simulink model "Half_Car_Model"  (R2024b)
settings: Solver=VariableStepAuto  StartTime=0.0  StopTime=4.5  RelTol=1e-3
model workspace (MAT data in the model file):
  I_yy = Simulink.Parameter
  I_yy.Value = 76.97
  I_yy.Complexity = 'real'
  I_yy.Dimensions = [1 1]
  I_yy.Description = 'Pitch moment of inertia (from solidworks TG19)'
  I_yy.DataType = 'auto'
  I_yy.DocUnits = 'kg/m/m'
  L = Simulink.Parameter
  L.Value = 1.49
  L.Complexity = 'real'
  L.Dimensions = [1 1]
  L.Description = 'wheelbase TG19 solidworks'
  L.DataType = 'auto'
  L.DocUnits = 'm'
  L_F = Simulink.Parameter
  L_F.Value = 0.91
  L_F.Complexity = 'real'
  L_F.Dimensions = [1 1]
  L_F.Description = 'distance from COM to front axle'
  L_F.DataType = 'auto'
  L_F.DocUnits = 'm'
  L_R = Simulink.Parameter
  L_R.Value = 0.58
  L_R.Complexity = 'real'
  L_R.Dimensions = [1 1]
  L_R.Description = 'distance from COM to rear axle'
  L_R.DataType = 'auto'
  L_R.DocUnits = 'm'
  c_Fs = Simulink.Parameter
  c_Fs.Value = 237.5
  c_Fs.Complexity = 'real'
  c_Fs.Dimensions = [1 1]
  c_Fs.Description = 'Shock damping from TG19 Spring Sheet'
  c_Fs.DataType = 'auto'
  c_Fs.DocUnits = 'kg/s'
  c_Fw = Simulink.Parameter
  c_Fw.Value = 1500
  c_Fw.Complexity = 'real'
  c_Fw.Dimensions = [1 1]
  c_Fw.Description = 'Tyre damping from Internet Value'
  c_Fw.DataType = 'auto'
  c_Fw.DocUnits = 'kg/s'
  c_Rs = Simulink.Parameter
  c_Rs.Value = 237.5
  c_Rs.Complexity = 'real'
  c_Rs.Dimensions = [1 1]
  c_Rs.Description = 'Shock damping from TG19 Spring Sheet'
  c_Rs.DataType = 'auto'
  c_Rs.DocUnits = 'kg/s'
  c_Rw = Simulink.Parameter
  c_Rw.Value = 1500
  c_Rw.Complexity = 'real'
  c_Rw.Dimensions = [1 1]
  c_Rw.Description = 'Tyre damping from Internet Value'
  c_Rw.DataType = 'auto'
  c_Rw.DocUnits = 'kg/s'
  gLong = Simulink.Parameter
  gLong.Value = 0
  gLong.Complexity = 'real'
  gLong.Dimensions = [1 1]
  gLong.Description = 'Longitudinal acceleration of car'
  gLong.DataType = 'auto'
  gLong.DocUnits = 'm/s/s'
  h = Simulink.Parameter
  h.Value = 0.51
  h.Complexity = 'real'
  h.Dimensions = [1 1]
  h.Description = 'height of com above ground at ride height (guessed)'
  h.DataType = 'auto'
  h.DocUnits = 'm'
  k_Fs = Simulink.Parameter
  k_Fs.Value = 3159.177
  k_Fs.Complexity = 'real'
  k_Fs.Dimensions = [1 1]
  k_Fs.Description = 'Shock Spring Rate from TG19 Shocks sheet (wheel rate value)'
  k_Fs.DataType = 'double'
  k_Fs.DocUnits = 'N/m'
  k_Fw = Simulink.Parameter
  k_Fw.Value = 30992
  k_Fw.Complexity = 'real'
  k_Fw.Dimensions = [1 1]
  k_Fw.Description = 'Tire Spring Stiffness (from internet value)'
  k_Fw.DataType = 'auto'
  k_Fw.DocUnits = 'N/m'
  k_Rs = Simulink.Parameter
  k_Rs.Value = 3159.177
  k_Rs.Complexity = 'real'
  k_Rs.Dimensions = [1 1]
  k_Rs.Description = 'Shock Spring Rate from TG19 Shocks sheet (wheel rate value)'
  k_Rs.DataType = 'double'
  k_Rs.DocUnits = 'N/m'
  k_Rw = Simulink.Parameter
  k_Rw.Value = 30992
  k_Rw.Complexity = 'real'
  k_Rw.Dimensions = [1 1]
  k_Rw.Description = 'Tire Spring Stiffness (from internet value)'
  k_Rw.DataType = 'auto'
  k_Rw.DocUnits = 'N/m'
  m_F = Simulink.Parameter
  m_F.Value = 27.27
  m_F.Complexity = 'real'
  m_F.Dimensions = [1 1]
  m_F.Description = 'Unsprung front axle mass'
  m_F.DataType = 'auto'
  m_F.DocUnits = 'kg'
  m_R = Simulink.Parameter
  m_R.Value = 27.7
  m_R.Complexity = 'real'
  m_R.Dimensions = [1 1]
  m_R.Description = 'unsprung rear axle mass from TG19 Shock sheet
    | = 30*2'
  m_R.DataType = 'auto'
  m_R.DocUnits = 'kg'
  m_s = Simulink.Parameter
  m_s.Value = 129
  m_s.Complexity = 'real'
  m_s.Dimensions = [1 1]
  m_s.Description = 'sprung mass from TG19 Shock sheet without 60kg driver'
  m_s.DataType = 'auto'
  m_s.DocUnits = 'kg'
  v = Simulink.Parameter
  v.Value = 11
  v.Complexity = 'real'
  v.Dimensions = [1 1]
  v.Description = 'initial velocity of car (40kph)'
  v.DataType = 'auto'
  v.DocUnits = 'm/s'
values from neighbouring files (symbols this model uses):
  L_F = mdlWks.getVariable('L_F').Value    [HCM_Animation.m]
  L_R = mdlWks.getVariable('L_R').Value    [HCM_Animation.m]
  v = -(amp/2)*freq*cos(freq*t)*.0254    [BumpBump.m]
libraries: simulink x1
settings Model: Creator=arnav  LastModifiedBy=arnav
settings RTWCC: GPUComputeCapability=3.5

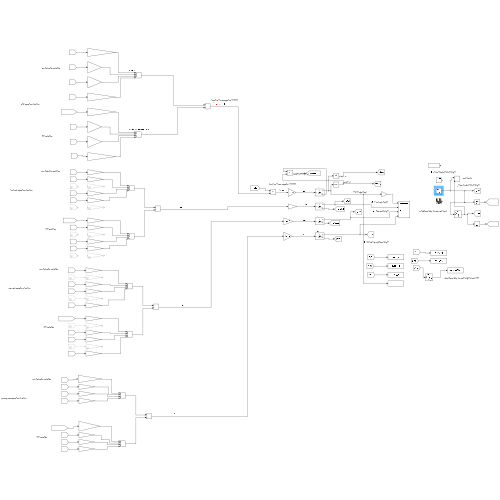
[thumbnail: Simulink's stored preview of the top-level diagram]
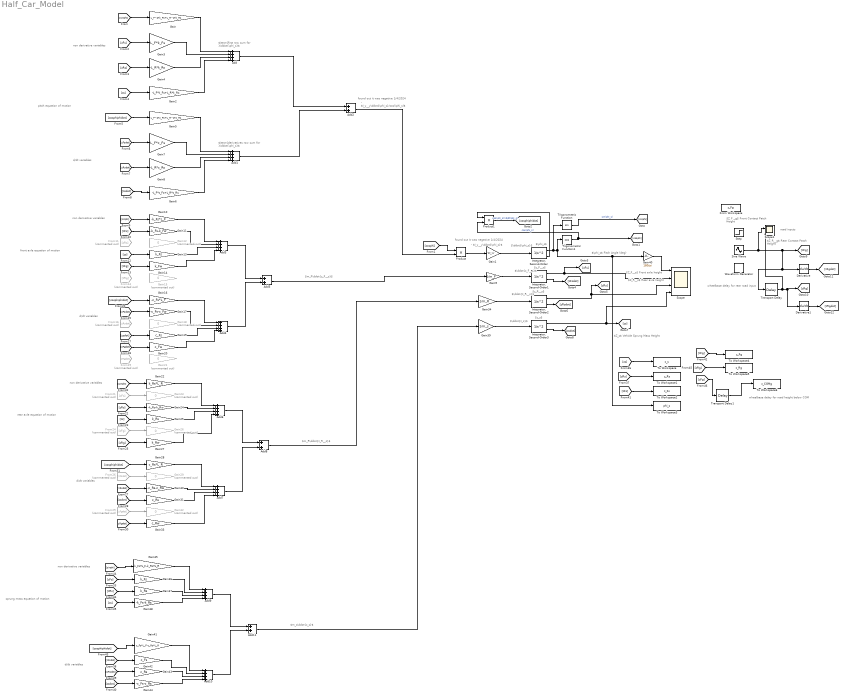
== system Half_Car_Model ==
  note: $Z_F__g$ Front Contact Patch Height
  note: found out it was negative 1/4/2024
  note: $Z_F__s$ Front axle height
  note: $m_F\ddot{z_F__s}$
  note: wheelbase delay for rear road input
  note: road inputs
  note: front axle equation of motion
  note: pitch equation of motion
  note: - $I_y__y\ddot{\phi_s}/cos(\phi_s)$
  note: $\text{first row sum for }\ddot{\phi_s}$
  note: $\phi_s$ Pitch Angle (deg)
  note: d/dt variables
  note: non derivative variables
  note: $z_s$
  note: $z_F__s$
  note: $\phi_s$
  note: $z_R__s$
  note: $\ddot{\phi_s}$
  note: - $I_y__y\ddot{\phi_s}$
  note: $\text{derivatives row sum for }\ddot{\phi_s}$
  note: $\ddot{z_F__s}$
  note: d/dt variables
  note: non derivative variables
  note: rear axle equation of motion
  note: d/dt variables
  note: non derivative variables
  note: $m_R\ddot{z_R__s}$
  note: $\ddot{z_R__s}$
  note: $m_s\ddot{z_s}$
  note: d/dt variables
  note: non derivative variables
  note: sprung mass equation of motion
  note: $\ddot{z_s}$
  note: $Z_R__s$ Rear axle height
  note: $Z_s$ Vehicle Sprung Mass Height
  note: found out it was negative 1/4/2024
  note: $Z_R__g$ Rear Contact Patch Height
  note: wheelbase delay for road height below COM
  Add{,1,3..4,6..7,9..10} (8 alike) : Sum  Inputs=++++
  Add{2,5,8,11} (4 alike) : Sum
  Derivative : Derivative
  Derivative1 : Derivative
  From Workspace : FromWorkspace  VariableName=z_Fg
  From11 : From  Commented=on  GotoTag=zRs
  From14 : From  Commented=on  GotoTag=zRg
  From16 : From  Commented=on  GotoTag=zRsdot
  From19 : From  Commented=on  GotoTag=zRgdot
  From21 : From  Commented=on  GotoTag=zFs
  From24 : From  Commented=on  GotoTag=zFg
  From26 : From  Commented=on  GotoTag=zFsdot
  From29 : From  Commented=on  GotoTag=zFgdot
  Gain : Gain  Gain=L_F^2*k_Fs+L_R^2*k_Rs
  Gain1 : Gain  Gain=-1/I_yy
  Gain10 : Gain  Gain=-k_Fs*L_F
  Gain11 : Gain  Gain=-k_Fs-k_Fw
  Gain{12,15,18,21,23,26,29,32} (8 alike) : Gain  Commented=on  Gain=0
  Gain13 : Gain  Gain=k_Fs
  Gain14 : Gain  Gain=k_Fw
  Gain16 : Gain  Gain=-c_Fs*L_F
  Gain17 : Gain  Gain=-c_Fs-c_Fw
  Gain19 : Gain  Gain=c_Fs
  Gain2 : Gain  Gain=-L_F*k_Fs+L_R*k_Rs
  Gain20 : Gain  Gain=c_Fw
  Gain22 : Gain  Gain=k_Rs*L_R
  Gain24 : Gain  Gain=-k_Rs-k_Rw
  Gain25 : Gain  Gain=k_Rs
  Gain27 : Gain  Gain=k_Rw
  Gain28 : Gain  Gain=c_Rs*L_R
  Gain3 : Gain  Gain=L_F*k_Fs
  Gain30 : Gain  Gain=-c_Rs-c_Rw
  Gain31 : Gain  Gain=c_Rs
  Gain33 : Gain  Gain=c_Rw
  Gain34 : Gain  Gain=1/m_R
  Gain35 : Gain  Gain=k_Fs*L_F-k_Rs*L_R
  Gain36 : Gain  Gain=k_Fs
  Gain37 : Gain  Gain=k_Rs
  Gain38 : Gain  Gain=-k_Fs-k_Rs
  Gain39 : Gain  Gain=1/m_s
  Gain4 : Gain  Gain=-L_R*k_Rs
  Gain40 : Gain  Gain=180/pi
  Gain41 : Gain  Gain=c_Fs*L_F-c_Rs*L_R
  Gain42 : Gain  Gain=c_Fs
  Gain43 : Gain  Gain=c_Rs
  Gain44 : Gain  Gain=-c_Fs-c_Rs
  Gain5 : Gain  Gain=L_F^2*c_Fs+L_R^2*c_Rs
  Gain6 : Gain  Gain=-L_F*c_Fs+L_R*c_Rs
  Gain7 : Gain  Gain=L_F*c_Fs
  Gain8 : Gain  Gain=-L_R*c_Rs
  Gain9 : Gain  Gain=1/m_F
  Integrator, Second-Order{,1..3} (4 alike) : SecondOrderIntegrator
  Product : Product
  Product1 : Product
  Scope : Scope  NumInputPorts=4
  Scope1 : Scope  NumInputPorts=2
  Sine Wave : Sin  Amplitude=0.2  Bias=0.2  Frequency=4  Phase=-pi/2  SampleTime=0
  Step : Step  After=0.3  SampleTime=0
  To Workspace : ToWorkspace  VariableName=z_s  SaveFormat=Timeseries  SampleTime=-1
  To Workspace1 : ToWorkspace  VariableName=z_Rs  SaveFormat=Timeseries  SampleTime=-1
  To Workspace2 : ToWorkspace  VariableName=z_Fs  SaveFormat=Timeseries  SampleTime=-1
  To Workspace3 : ToWorkspace  VariableName=phi_s  SaveFormat=Timeseries  SampleTime=-1
  To Workspace4 : ToWorkspace  VariableName=z_Fg  SaveFormat=Timeseries  SampleTime=-1
  To Workspace5 : ToWorkspace  VariableName=z_Rg  SaveFormat=Timeseries  SampleTime=-1
  To Workspace6 : ToWorkspace  VariableName=z_COMg  SaveFormat=Timeseries  SampleTime=-1
  Transport Delay : TransportDelay  DelayTime=L/v
  Transport Delay1 : TransportDelay  DelayTime=L_F/v
  Trigonometric Function : Trigonometry
  Trigonometric Function1 : Trigonometry  Operator=cos
  Waveform Generator : simulink/Sources/Waveform Generator  OutMin=[]  OutMax=[]  OutDataTypeStr=double  SelectedSignal=1  Signals=0#  BlockNames=MultiportSwitch_dade414a57e3400#MultiportSwitch_f75317cf24ba448  SampleTime=0.1
  wires:
  "Integrator, Second-Order1"/1 -> Scope/2, [zFs]
  "Integrator, Second-Order2"/1 -> [zRs], Scope/3
  "Integrator, Second-Order3"/1 -> Scope/4, [zs]
  Trigonometric Function/1 -> [sinphi]  "sin(phi_s)"
  Trigonometric Function1/1 -> Product1/2, [cosphi]  "cos(phi_s)"
  Product/1 -> Gain1/1
  Gain1/1 -> "Integrator, Second-Order"/1
  Add2/1 -> Product/2
  "Integrator, Second-Order"/2 -> Product1/1
  Product1/1 -> [cosphiphidot]  "cos(phi_s)*d/dt(phi_s)"
  [cosphi] -> Product/1
  "Integrator, Second-Order1"/2 -> [zFsdot]
  "Integrator, Second-Order2"/2 -> [zRsdot]
  "Integrator, Second-Order3"/2 -> [zsdot]
  [sinphi] -> Gain/1
  [zFs] -> Gain3/1
  [zRs] -> Gain4/1
  [zs] -> Gain2/1
  Gain/1 -> Add/1
  Gain3/1 -> Add/2
  Gain4/1 -> Add/3
  Gain2/1 -> Add/4
  Add/1 -> Add2/1
  Gain8/1 -> Add1/3
  Gain6/1 -> Add1/4
  Gain5/1 -> Add1/1
  Add1/1 -> Add2/2
  Gain7/1 -> Add1/2
  [cosphiphidot] -> Gain5/1
  [zFsdot] -> Gain7/1
  [zRsdot] -> Gain8/1
  [zsdot] -> Gain6/1
  Gain9/1 -> "Integrator, Second-Order1"/1
  Derivative/1 -> [zFgdot]
  Derivative1/1 -> [zRgdot]
  Sine Wave/1 -> Scope1/1, Transport Delay/1, Derivative/1, [zFg]
  Transport Delay/1 -> Scope1/2, Derivative1/1, [zRg]
  [sinphi] -> Gain10/1
  [zFs] -> Gain11/1
  [zs] -> Gain13/1
  [zFg] -> Gain14/1
  Gain10/1 -> Add3/1
  Gain11/1 -> Add3/2
  Gain13/1 -> Add3/3
  Gain14/1 -> Add3/4
  [zsdot] -> Gain19/1
  [cosphiphidot] -> Gain16/1
  Gain19/1 -> Add4/3
  Gain16/1 -> Add4/1
  [zFsdot] -> Gain17/1
  Gain20/1 -> Add4/4
  Gain17/1 -> Add4/2
  [zFgdot] -> Gain20/1
  Add3/1 -> Add5/1
  Add4/1 -> Add5/2
  Add5/1 -> Gain9/1
  Add8/1 -> Gain34/1
  From21/1 -> Gain23/1
  Gain22/1 -> Add6/1
  From29/1 -> Gain32/1
  [zsdot] -> Gain31/1
  Gain31/1 -> Add7/3
  Gain28/1 -> Add7/1
  From26/1 -> Gain29/1
  [zs] -> Gain25/1
  [sinphi] -> Gain22/1
  From24/1 -> Gain26/1
  Gain25/1 -> Add6/3
  [cosphiphidot] -> Gain28/1
  Add7/1 -> Add8/2
  Add6/1 -> Add8/1
  Gain24/1 -> Add6/2
  Gain27/1 -> Add6/4
  Gain30/1 -> Add7/2
  Gain33/1 -> Add7/4
  Gain34/1 -> "Integrator, Second-Order2"/1
  [sinphi] -> Gain35/1
  Gain35/1 -> Add9/1
  Gain43/1 -> Add10/3
  Gain41/1 -> Add10/1
  Gain44/1 -> Add10/4
  Gain38/1 -> Add9/4
  [zsdot] -> Gain44/1
  [zFsdot] -> Gain42/1
  [cosphiphidot] -> Gain41/1
  [zFs] -> Gain36/1
  Gain37/1 -> Add9/3
  Add9/1 -> Add11/1
  Add10/1 -> Add11/2
  Add11/1 -> Gain39/1
  [zs] -> Gain38/1
  Gain42/1 -> Add10/2
  Gain36/1 -> Add9/2
  Gain39/1 -> "Integrator, Second-Order3"/1
  [zRs] -> Gain24/1
  [zRg] -> Gain27/1
  [zRsdot] -> Gain30/1
  [zRgdot] -> Gain33/1
  [zRs] -> Gain37/1
  [zRsdot] -> Gain43/1
  Gain40/1 -> Scope/1
  [zs] -> To Workspace/1
  [zRs] -> To Workspace1/1
  [zFs] -> To Workspace2/1
  "Integrator, Second-Order"/1 -> Trigonometric Function/1, Gain40/1, To Workspace3/1, Trigonometric Function1/1
  [zFg] -> To Workspace4/1
  [zRg] -> To Workspace5/1
  [zFg] -> Transport Delay1/1
  Transport Delay1/1 -> To Workspace6/1
